simulink model "Montagem_ServoSimples"  (Simulink 7.2)
settings: Solver=ode45  StartTime=0.0  StopTime=10.0  RelTol=1e-3
undefined symbols (not defined in the file): RootGround, RootPart, Servo_Simples, ServoHornPlastic
libraries: mblibv1 x8
settings Model: Creator=LAraujo  LastModifiedBy=LAraujo
settings SimMechanicsCC: VisOnUpdateDiagram=on  VisDuringSimulation=on

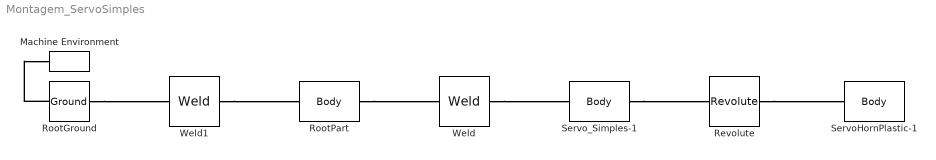
== system Montagem_ServoSimples ==
  Machine Environment : mblibv1/Bodies/Machine Environment  Orientation=left  DialogController=MECH.DialogSource  SystemSampleTime=-1  PortType=env  PhysicalDomain=Mechanical  DialogTemplateClass=MECH.MachineEnvironment  SyncWhenCopied=off  Gravity=[0 -9.81 0]  GravityUnits=m/s^2  GravityAsSignal=off  Dimensionality=Auto-detect  AnalysisType=Forward dynamics  LinearAssemblyTolerance=1e-3  LinearAssemblyToleranceUnits=m  AngularAssemblyTolerance=1e-3  AngularAssemblyToleranceUnits=rad  ConstraintSolverType=Stabilizing  ConstraintRelTolerance=1e-4  ConstraintAbsTolerance=1e-4  UseRobustSingularityHandling=off  RedundancyAnalysisToleranceType=Automatically select tolerance  RedundancyAnalysisTolerance=1e-14  StatePerturbationType=Fixed  PerturbationSize=1e-5  VisualizeMachine=on  BodyVisualizationType=Use model default body geometries  BodyColorSelMode=Use model default  DefaultBodyColor=[1 0 0]
  Revolute : mblibv1/Joints/Revolute  DialogController=MECH.DynMechDlgSource  PhysicalDomain=mechanical  SubClassName=Unknown  LeftPortType=blob  RightPortType=blob  LConnTagsString=__newl0  RConnTagsString=__newr0  PMImportedID=ServoHornPlastic-1:-:Servo_Simples-1  UpdateFromCAD=on  NumSAPorts=0  CutJoint=off  MarkAsCut=off  Primitives=prismatic  PrimitiveProps=R1$WORLD$[0,0,1]$revolute  DialogClass=JointBlock  R1Axis=[0,0,1]
  RootGround : mblibv1/Bodies/Ground  DialogController=MECH.DynMechDlgSource  SystemSampleTime=-1  PMImportedID=RootGround  UpdateFromCAD=on  LeftPortType=env  RightPortType=workingframe  PhysicalDomain=Mechanical  DialogClass=GroundBlock  CoordPosition=[-0.00325605,0.000392966,-0.00120744]  CoordPositionUnits=m  StateVectorMgrId=1  MachineId=[2 0]  ShowEnvPort=on
  RootPart : mblibv1/Bodies/Body  DialogController=MECH.DynMechDlgSource  PhysicalDomain=mechanical  SubClassName=Unknown  LeftPortType=workingframe  RightPortType=workingframe  LConnTagsString=CS3  RConnTagsString=CS2  PMImportedID=RootPart  UpdateFromCAD=on  DialogClass=MechanicalBodyBlock  Mass=0  MassUnits=kg  InertiaUnits=kg*m^2  Inertia=[0,0,0;0,0,0;0,0,0]  Shape=Cylinder  ShapeDims=[1 1]  ShapeUnits=m  ShapeUse=false  Density=1  DensityUnits=kg/m^3  DensityUse=false  GraphicsMode=MACHINE_DEFAULT  BodyColorSelMode=MACHINE_DEFAULT  BodyColor=[1 0 0]  AttachedToCS=CS1  CG=Right$CG$[-0.00325605 0.000392966 -0.00120744]$WORLD$WORLD$m$[1 0 0;0 1 0;0 0 1]$3x3 Transform$rad$WORLD$false$RootPart::CG(AUTOGEN)  WorkingFrames=Right$CS1$[0 0 0]$WORLD$WORLD$m$[1 0 0;0 1 0;0 0 1]$3x3 Transform$rad$WORLD$false$RootPart::CS1(AUTOGEN)#Right$CS2$[-0.00331151 0.00039206 -0.00109331]$WORLD$WORLD$m$[1 0 0;0 1 0;0 0 1]$3x3 Transform$rad$WORLD$true$RootPart:-:Servo_Simples-1::RootPart(AUTOGEN)#Left$CS3$[-0.00325605 0.000392966 -0.00120744]$WORLD$WORLD$m$[1 0 0;0 1 0;0 0 1]$3x3 Transform$rad$WORLD$true$RootGround:-:RootPart::RootPart(AUTOGEN)  CGPos=[-0.00325605 0.000392966 -0.00120744]  CGRot=[1 0 0;0 1 0;0 0 1]  CS0Pos=[]  CS0Rot=[]  CS1Pos=[0 0 0]  CS1Rot=[1 0 0;0 1 0;0 0 1]  CS2Pos=[-0.00331151 0.00039206 -0.00109331]  CS2Rot=[1 0 0;0 1 0;0 0 1]  CS3Pos=[-0.00325605 0.000392966 -0.00120744]  CS3Rot=[1 0 0;0 1 0;0 0 1]  CS4Pos=[]  CS4Rot=[]  CS5Pos=[]  CS5Rot=[]  CS6Pos=[]  CS6Rot=[]  CS7Pos=[]  CS7Rot=[]  CS8Pos=[]  CS8Rot=[]  CS9Pos=[]  CS9Rot=[]  CS10Pos=[]  CS10Rot=[]  CS11Pos=[]  CS11Rot=[]  CS12Pos=[]  CS12Rot=[]  CS13Pos=[]  CS13Rot=[]  CS14Pos=[]  CS14Rot=[]  CS15Pos=[]  CS15Rot=[]  CS16Pos=[]  CS16Rot=[]  CS17Pos=[]  CS17Rot=[]  CS18Pos=[]  CS18Rot=[]  CS19Pos=[]  CS19Rot=[]  CS20Pos=[]  CS20Rot=[]
  ServoHornPlastic-1 : mblibv1/Bodies/Body  DialogController=MECH.DynMechDlgSource  PhysicalDomain=mechanical  SubClassName=Unknown  LeftPortType=workingframe  RightPortType=workingframe  LConnTagsString=CS2  PMImportedID=ServoHornPlastic-1  UpdateFromCAD=on  DialogClass=MechanicalBodyBlock  Mass=0.00107043  MassUnits=kg  InertiaUnits=kg*m^2  Inertia=[3.77224e-008,0,0;0,7.26212e-008,0;0,0,3.65964e-008]  Shape=Cylinder  ShapeDims=[1 1]  ShapeUnits=m  ShapeUse=false  Density=1  DensityUnits=kg/m^3  DensityUse=false  GraphicsMode=GFXFILE  GraphicsFileName=Montagem_ServoSimples - ServoHornPlastic-1.STL  BodyColorSelMode=COLORPALETTE  BodyColor=[0.698039;0.698039;0.698039]  AttachedToCS=CS1  CG=Right$CG$[0.00667762 0.000555315 -0.0216488]$WORLD$WORLD$m$[0.999756 0 -0.0220735;0.0220735 0 0.999756;0 -1 0]$3x3 Transform$rad$WORLD$false$ServoHornPlastic-1::CG(AUTOGEN)  WorkingFrames=Right$CS1$[0.00667762 0.000555315 -0.02285]$WORLD$WORLD$m$[0.999756 0 -0.0220735;0.0220735 0 0.999756;0 -1 0]$3x3 Transform$rad$WORLD$false$ServoHornPlastic-1::CS1(AUTOGEN)#Left$CS2$[0.00667762 0.000555315 -0.02135]$WORLD$WORLD$m$[1 0 0;0 1 0;0 0 1]$3x3 Transform$rad$WORLD$true$ServoHornPlastic-1:-:Servo_Simples-1::ServoHornPlastic-1(AUTOGEN)  CGPos=[0.00667762 0.000555315 -0.0216488]  CGRot=[0.999756 0 -0.0220735;0.0220735 0 0.999756;0 -1 0]  CS0Pos=[]  CS0Rot=[]  CS1Pos=[0.00667762 0.000555315 -0.02285]  CS1Rot=[0.999756 0 -0.0220735;0.0220735 0 0.999756;0 -1 0]  CS2Pos=[0.00667762 0.000555315 -0.02135]  CS2Rot=[1 0 0;0 1 0;0 0 1]  CS3Pos=[]  CS3Rot=[]  CS4Pos=[]  CS4Rot=[]  CS5Pos=[]  CS5Rot=[]  CS6Pos=[]  CS6Rot=[]  CS7Pos=[]  CS7Rot=[]  CS8Pos=[]  CS8Rot=[]  CS9Pos=[]  CS9Rot=[]  CS10Pos=[]  CS10Rot=[]  CS11Pos=[]  CS11Rot=[]  CS12Pos=[]  CS12Rot=[]  CS13Pos=[]  CS13Rot=[]  CS14Pos=[]  CS14Rot=[]  CS15Pos=[]  CS15Rot=[]  CS16Pos=[]  CS16Rot=[]  CS17Pos=[]  CS17Rot=[]  CS18Pos=[]  CS18Rot=[]  CS19Pos=[]  CS19Rot=[]  CS20Pos=[]  CS20Rot=[]
  Servo_Simples-1 : mblibv1/Bodies/Body  DialogController=MECH.DynMechDlgSource  PhysicalDomain=mechanical  SubClassName=Unknown  LeftPortType=workingframe  RightPortType=workingframe  LConnTagsString=CS2  RConnTagsString=CS3  PMImportedID=Servo_Simples-1  UpdateFromCAD=on  DialogClass=MechanicalBodyBlock  Mass=0.191711  MassUnits=kg  InertiaUnits=kg*m^2  Inertia=[2.66902e-005,-2.21506e-009,-3.18594e-007;-2.21506e-009,4.55319e-005,9.87505e-009;-3.18594e-007,9.87505e-009,3.14869e-005]  Shape=Cylinder  ShapeDims=[1 1]  ShapeUnits=m  ShapeUse=false  Density=1  DensityUnits=kg/m^3  DensityUse=false  GraphicsMode=GFXFILE  GraphicsFileName=Montagem_ServoSimples - Servo_Simples-1.STL  BodyColorSelMode=COLORPALETTE  BodyColor=[0.231373;0.231373;0.231373]  AttachedToCS=CS1  CG=Right$CG$[-0.00331151 0.00039206 -0.00109331]$WORLD$WORLD$m$[1 0 0;0 1 0;0 0 1]$3x3 Transform$rad$WORLD$false$Servo_Simples-1::CG(AUTOGEN)  WorkingFrames=Right$CS1$[0.00672906 -0.00941128 -1.65475e-014]$WORLD$WORLD$m$[1 0 0;0 1 0;0 0 1]$3x3 Transform$rad$WORLD$false$Servo_Simples-1::CS1(AUTOGEN)#Left$CS2$[-0.00331151 0.00039206 -0.00109331]$WORLD$WORLD$m$[1 0 0;0 1 0;0 0 1]$3x3 Transform$rad$WORLD$true$RootPart:-:Servo_Simples-1::Servo_Simples-1(AUTOGEN)#Right$CS3$[0.00667762 0.000555315 -0.02135]$WORLD$WORLD$m$[1 0 0;0 1 0;0 0 1]$3x3 Transform$rad$WORLD$true$ServoHornPlastic-1:-:Servo_Simples-1::Servo_Simples-1(AUTOGEN)  CGPos=[-0.00331151 0.00039206 -0.00109331]  CGRot=[1 0 0;0 1 0;0 0 1]  CS0Pos=[]  CS0Rot=[]  CS1Pos=[0.00672906 -0.00941128 -1.65475e-014]  CS1Rot=[1 0 0;0 1 0;0 0 1]  CS2Pos=[-0.00331151 0.00039206 -0.00109331]  CS2Rot=[1 0 0;0 1 0;0 0 1]  CS3Pos=[0.00667762 0.000555315 -0.02135]  CS3Rot=[1 0 0;0 1 0;0 0 1]  CS4Pos=[]  CS4Rot=[]  CS5Pos=[]  CS5Rot=[]  CS6Pos=[]  CS6Rot=[]  CS7Pos=[]  CS7Rot=[]  CS8Pos=[]  CS8Rot=[]  CS9Pos=[]  CS9Rot=[]  CS10Pos=[]  CS10Rot=[]  CS11Pos=[]  CS11Rot=[]  CS12Pos=[]  CS12Rot=[]  CS13Pos=[]  CS13Rot=[]  CS14Pos=[]  CS14Rot=[]  CS15Pos=[]  CS15Rot=[]  CS16Pos=[]  CS16Rot=[]  CS17Pos=[]  CS17Rot=[]  CS18Pos=[]  CS18Rot=[]  CS19Pos=[]  CS19Rot=[]  CS20Pos=[]  CS20Rot=[]
  Weld : mblibv1/Joints/Weld  DialogController=MECH.DynMechDlgSource  PhysicalDomain=mechanical  SubClassName=Unknown  LeftPortType=blob  RightPortType=blob  LConnTagsString=__newl0  RConnTagsString=__newr0  PMImportedID=RootPart:-:Servo_Simples-1  UpdateFromCAD=on  NumSAPorts=0  CutJoint=off  MarkAsCut=off  Primitives=weld  PrimitiveProps=W$WORLD$[0.57735,0.57735,0.57735]$weld  DialogClass=JointBlock  WAxis=[0.57735,0.57735,0.57735]
  Weld1 : mblibv1/Joints/Weld  DialogController=MECH.DynMechDlgSource  PhysicalDomain=mechanical  SubClassName=Unknown  LeftPortType=blob  RightPortType=blob  LConnTagsString=__newl0  RConnTagsString=__newr0  PMImportedID=RootGround:-:RootPart  UpdateFromCAD=on  NumSAPorts=0  CutJoint=off  MarkAsCut=off  Primitives=weld  PrimitiveProps=W$WORLD$[0.57735,0.57735,0.57735]$weld  DialogClass=JointBlock  WAxis=[0.57735,0.57735,0.57735]
  connections:
  RootPart/RConn1 -- Weld/LConn1
  Weld/RConn1 -- Servo_Simples-1/LConn1
  Servo_Simples-1/RConn1 -- Revolute/LConn1
  Revolute/RConn1 -- ServoHornPlastic-1/LConn1
  RootGround/RConn1 -- Weld1/LConn1
  Weld1/RConn1 -- RootPart/LConn1
  RootGround/LConn1 -- Machine Environment/RConn1
